simulink model "prova_LOG_DATI_07_13"  (R2020b)
settings: Solver=VariableStepAuto  StartTime=0.0  StopTime=inf  RelTol=1e-3
values from neighbouring files (symbols this model uses):
  t_AP = 0.02    [AVVIO_YAK_DATA.m]
libraries: simulink_extras x12, svdutilitieslib x2
settings Model: Creator=alexv  LastModifiedBy=lapis-dspace

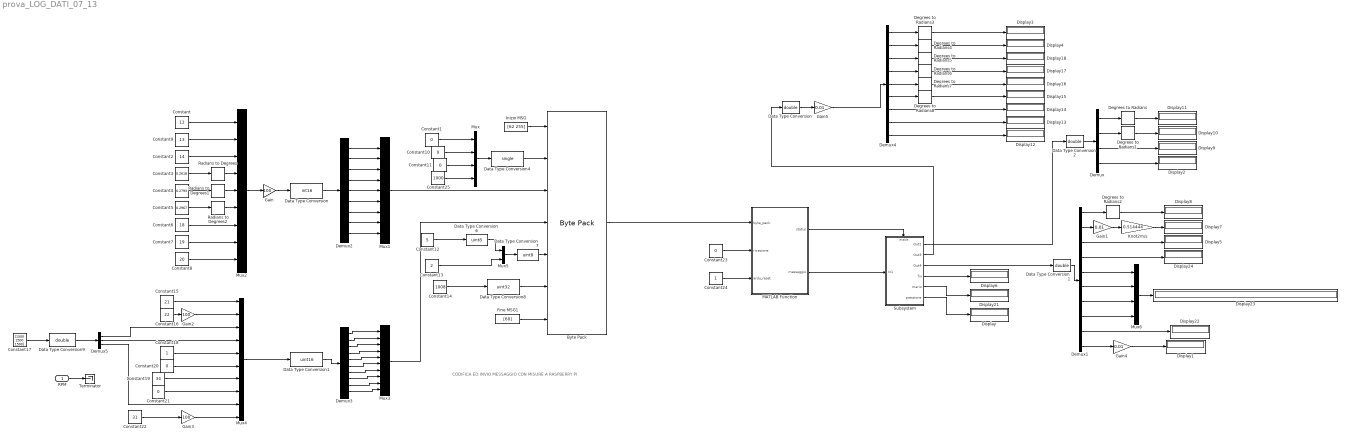
== system prova_LOG_DATI_07_13 ==
  note: CODIFICA ED INVIO MESSAGGIO CON MISURE A RASPBERRY PI
  RPM : Inport
  Byte Pack : svdutilitieslib/Byte Pack  maskPackedDataType=uint8  datatypes={'uint8','single','int16','uint16','uint8','uint32','uint8'}  byteAlign=1  blockPlatform=arduinoert
      settings: SourceProductBaseCode=ARDUINO
  Constant : Constant  Value=12
  Constant{1,10..11,20..21,23} (6 alike) : Constant  Value=0
  Constant12 : Constant  Value=5
  Constant13 : Constant  Value=2  OutDataTypeStr=uint8
  Constant14 : Constant  Value=1008  SampleTime=0.02
  Constant15 : Constant  Value=21
  Constant16 : Constant  Value=22
  Constant17 : Constant  Value="[1500  1500 1500]"
  Constant18 : Constant
  Constant19 : Constant  Value=34
  Constant2 : Constant  Value=14
  Constant22 : Constant  Value=31  SampleTime=0.02
  Constant24 : Constant
  Constant25 : Constant  Value=1000
  Constant3 : Constant  Value=0.2618
  Constant4 : Constant  Value=0.2793
  Constant5 : Constant  Value=0.2967
  Constant6 : Constant  Value=18
  Constant7 : Constant  Value=19
  Constant8 : Constant  Value=20
  Constant9 : Constant  Value=13
  Data Type Conversion{,1..2,9} (4 alike) : DataTypeConversion  OutDataTypeStr=double
  Data Type Conversion : DataTypeConversion  OutDataTypeStr=int16
  Data Type Conversion1 : DataTypeConversion  OutDataTypeStr=uint16
  Data Type Conversion4 : DataTypeConversion  OutDataTypeStr=single
  Data Type Conversion6 : DataTypeConversion  OutDataTypeStr=uint8
  Data Type Conversion7 : DataTypeConversion  OutDataTypeStr=uint8
  Data Type Conversion8 : DataTypeConversion  OutDataTypeStr=uint32
  Degrees to Radians{,1..8} (9 alike) : simulink_extras/Transformations/Degrees to Radians
  Demux : Demux
  Demux1 : Demux  Outputs=10
  Demux2 : Demux  Outputs=9
  Demux3 : Demux  Outputs=10
  Demux4 : Demux  Outputs=9
  Demux5 : Demux  Outputs=3
  Display{,1..18,21..24} (23 alike) : Display
  Fine MSG1 : Constant  Value=[60]  OutDataTypeStr=uint8  SampleTime=t_AP
  Gain : Gain  Gain=100  OutDataTypeStr=single
  Gain1 : Gain  Gain=0.01
  Gain2 : Gain  Gain=100
  Gain3 : Gain  Gain=100  OutDataTypeStr=double
  Gain4 : Gain  Gain=0.01
  Gain5 : Gain  Gain=0.01
  Inizio MSG : Constant  Value=[62 255]  OutDataTypeStr=uint8  SampleTime=t_AP
  Knot2m/s : Gain  Gain=0.514444
  MATLAB Function : MATLAB Function  TreatAsAtomicUnit=on
  Mux : Mux
  Mux1 : Mux  Inputs=9
  Mux2 : Mux  Inputs=9
  Mux3 : Mux  Inputs=10
  Mux4 : Mux  Inputs=10
  Mux5 : Mux  Inputs=2
  Mux6 : Mux
  Radians to Degrees : simulink_extras/Transformations/Radians to Degrees
  Radians to Degrees1 : simulink_extras/Transformations/Radians to Degrees
  Radians to Degrees2 : simulink_extras/Transformations/Radians to Degrees
  Subsystem : Subsystem
  Terminator : Terminator
  wires:
  Demux5/3 -> Mux4/9
  Constant13/1 -> Mux5/2
  Demux2/7 -> Mux1/7
  RPM/1 -> Terminator/1
  Gain3/1 -> Mux4/10
  Constant9/1 -> Mux2/2
  Constant17/1 -> Data Type Conversion9/1
  Mux1/1 -> Byte Pack/3
  Constant14/1 -> Data Type Conversion8/1
  Mux2/1 -> Gain/1
  Demux3/9 -> Mux3/9
  Fine MSG1/1 -> Byte Pack/7
  Demux3/4 -> Mux3/4
  Data Type Conversion4/1 -> Byte Pack/2
  Constant12/1 -> Data Type Conversion6/1
  Data Type Conversion7/1 -> Byte Pack/5
  Data Type Conversion6/1 -> Mux5/1
  Constant/1 -> Mux2/1
  Data Type Conversion8/1 -> Byte Pack/6
  Demux3/8 -> Mux3/8
  Radians to Degrees1/1 -> Mux2/5
  Mux/1 -> Data Type Conversion4/1
  Constant22/1 -> Gain3/1
  Constant25/1 -> Mux/4
  Radians to Degrees/1 -> Mux2/4
  Gain2/1 -> Mux4/2
  Constant6/1 -> Mux2/7
  Constant2/1 -> Mux2/3
  Constant4/1 -> Radians to Degrees1/1
  Constant5/1 -> Radians to Degrees2/1
  Demux3/6 -> Mux3/6
  Mux3/1 -> Byte Pack/4
  Constant21/1 -> Mux4/8
  Data Type Conversion1/1 -> Demux3/1
  Demux5/1 -> Mux4/3
  Constant7/1 -> Mux2/8
  Constant8/1 -> Mux2/9
  Demux2/9 -> Mux1/9
  Demux3/3 -> Mux3/3
  Demux3/2 -> Mux3/2
  Demux3/7 -> Mux3/7
  Constant20/1 -> Mux4/6
  Data Type Conversion9/1 -> Demux5/1
  Demux3/5 -> Mux3/5
  Mux4/1 -> Data Type Conversion1/1
  Constant16/1 -> Gain2/1
  Constant18/1 -> Mux4/5
  Demux5/2 -> Mux4/4
  Inizio MSG/1 -> Byte Pack/1
  Demux2/2 -> Mux1/2
  Constant3/1 -> Radians to Degrees/1
  Demux2/1 -> Mux1/1
  Demux2/5 -> Mux1/5
  Radians to Degrees2/1 -> Mux2/6
  Constant10/1 -> Mux/2
  Demux3/10 -> Mux3/10
  Demux2/6 -> Mux1/6
  Demux2/4 -> Mux1/4
  Demux2/8 -> Mux1/8
  Constant11/1 -> Mux/3
  Data Type Conversion/1 -> Demux2/1
  Gain/1 -> Data Type Conversion/1
  Demux3/1 -> Mux3/1
  Mux5/1 -> Data Type Conversion7/1
  Constant1/1 -> Mux/1
  Constant19/1 -> Mux4/7
  Demux2/3 -> Mux1/3
  Constant15/1 -> Mux4/1
  Constant24/1 -> MATLAB Function/3(ardu_reset)
  Subsystem/6(pressione) -> Display/1
  Constant23/1 -> MATLAB Function/2(ricezione)
  MATLAB Function/2(messaggio) -> Subsystem/1(In1)
  Subsystem/3(Out4) -> Data Type Conversion1/1
  Subsystem/5(mario) -> Display21/1
  Byte Pack/1 -> MATLAB Function/1(byte_pack)
  MATLAB Function/1(status) -> Subsystem/Enable
  Subsystem/4("fix ") -> Display6/1
  Gain4/1 -> Display1/1
  Demux1/4 -> Display24/1
  Demux1/9 -> Display22/1
  Demux1/3 -> Display5/1
  Demux1/8 -> Mux6/4
  Demux1/10 -> Gain4/1
  Mux6/1 -> Display23/1
  Demux1/2 -> Gain1/1
  Demux1/6 -> Mux6/2
  Knot2m/s/1 -> Display7/1
  Gain1/1 -> Knot2m/s/1
  Data Type Conversion1/1 -> Demux1/1
  Demux1/7 -> Mux6/3
  Demux1/5 -> Mux6/1
  Demux1/1 -> Degrees to Radians2/1
  Degrees to Radians2/1 -> Display8/1
  Demux/1 -> Degrees to Radians/1
  Data Type Conversion2/1 -> Demux/1
  Subsystem/1(Out2) -> Data Type Conversion2/1
  Degrees to Radians/1 -> Display11/1
  Demux/3 -> Display9/1
  Demux/4 -> Display2/1
  Demux/2 -> Degrees to Radians1/1
  Degrees to Radians1/1 -> Display10/1
  Gain5/1 -> Demux4/1
  Data Type Conversion/1 -> Gain5/1
  Subsystem/2(Out3) -> Data Type Conversion/1
  Demux4/4 -> Degrees to Radians6/1
  Demux4/9 -> Display12/1
  Demux4/8 -> Display13/1
  Demux4/1 -> Degrees to Radians3/1
  Demux4/3 -> Degrees to Radians5/1
  Degrees to Radians3/1 -> Display3/1
  Demux4/2 -> Degrees to Radians4/1
  Demux4/6 -> Degrees to Radians8/1
  Degrees to Radians7/1 -> Display16/1
  Degrees to Radians8/1 -> Display15/1
  Degrees to Radians4/1 -> Display4/1
  Demux4/5 -> Degrees to Radians7/1
  Degrees to Radians5/1 -> Display18/1
  Demux4/7 -> Display14/1
  Degrees to Radians6/1 -> Display17/1

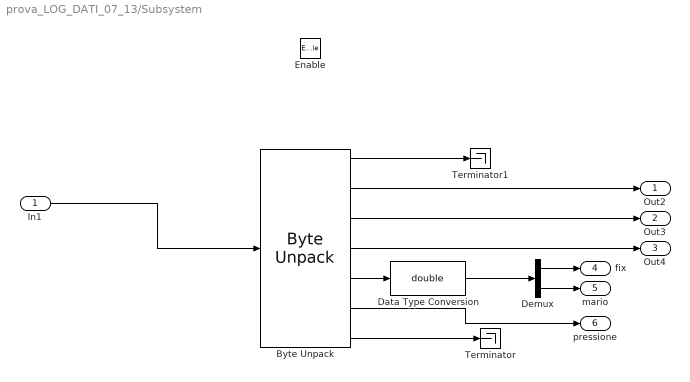
== system prova_LOG_DATI_07_13/Subsystem ==
  In1 : Inport
  Enable : EnablePort
  Byte Unpack : svdutilitieslib/Byte Unpack  dimensions={[2],[4],[9],[10],[2],[1],[1]}  datatypes={'uint8','single','int16','uint16','uint8','uint32','uint8'}  byteAlign=1  blockPlatform=arduinoert
      settings: SourceProductBaseCode=ARDUINO
  Data Type Conversion : DataTypeConversion  OutDataTypeStr=double
  Demux : Demux  Outputs=2
  Terminator : Terminator
  Terminator1 : Terminator
  Out2 : Outport  VectorParamsAs1DForOutWhenUnconnected=off
  Out3 : Outport  Port=2  VectorParamsAs1DForOutWhenUnconnected=off
  Out4 : Outport  Port=3  VectorParamsAs1DForOutWhenUnconnected=off
  "fix " : Outport  Port=4  VectorParamsAs1DForOutWhenUnconnected=off
  mario : Outport  Port=5  VectorParamsAs1DForOutWhenUnconnected=off
  pressione : Outport  Port=6  VectorParamsAs1DForOutWhenUnconnected=off
  wires:
  In1/1 -> Byte Unpack/1
  Byte Unpack/1 -> Terminator1/1
  Byte Unpack/4 -> Out4/1
  Byte Unpack/3 -> Out3/1
  Byte Unpack/2 -> Out2/1
  Byte Unpack/7 -> Terminator/1
  Byte Unpack/5 -> Data Type Conversion/1
  Demux/1 -> "fix "/1
  Demux/2 -> mario/1
  Data Type Conversion/1 -> Demux/1
  Byte Unpack/6 -> pressione/1

== matlab function prova_LOG_DATI_07_13/MATLAB Function ==
  data: byte_pack input; status output; messaggio output; ricezione input; ardu_reset input
function [status,messaggio]  = LETTURA_Arduino_mex(byte_pack,ricezione,ardu_reset)

persistent message counter start_found

status = false;                                        %ho aggiunto questo
messaggio = uint8(zeros(1,63)) ;
M = uint8(length(byte_pack)) ;
entrata = true ;

if isempty(start_found) 
     start_found = false ;
end 
if isempty (counter) 
    counter = uint8(0) ;
end 
if isempty(message)
     message = uint8(zeros(1,63)) ;
end

if ((ricezione ~= 0) || (ardu_reset == 0))
    start_found = false ;
    message = uint8(zeros(1,63)) ;
    counter = uint8(0)  ;
    entrata = false ;
end

if (start_found == 0 && entrata == true )
    for i = 1 : M-1  
        if ( byte_pack(i) == 62 &&  byte_pack(i + 1) == 255 )                  % mi conviene mandare un secondo byte all'inizio cosi non devo cambiare nulla
            message(1:M - (i-1)) = byte_pack(i:end) ;
            counter = M - (i-1) ; 
            start_found = true ;
            break
        end
    end   % lho messo qua
        if counter == M 
            messaggio = message ;
            message = uint8(zeros(1,63)) ;
            status = true ;
            start_found = false ;
            counter = uint8(0) ;
        end
     %end
    
    
elseif start_found == 1 

        message(counter + 1 : end) = byte_pack(1:M - counter) ;
        status = true;       %ho aggiunto questo
        messaggio = message ;
        counter = M - counter ;
        message = uint8(zeros(1,63)) ;
        
            for i = counter : M-1  
        if ( byte_pack(i) == 62 &&  byte_pack(i + 1) == 255 )                  % mi conviene mandare un secondo byte all'inizio cosi non devo cambiare nulla
            message(1:M - (i-1)) = byte_pack(i:end) ;
            counter = M - (i-1) ; 
            start_found = true ;
            break
        else 
            start_found = false ;
            counter = uint8(0);
        end 
            end
        
     %   message (1 : M-counter ) = byte_pack(counter + 1:end) ;
     %   counter = M - counter ;

end
